simulink model "Ring_modulator"  (Simulink 10.0)
settings: Solver=ode45  StartTime=0.0  StopTime=10.0  RelTol=1e-3  EnableMultiTasking=on
settings Model: Creator=tjohnson  LastModifiedBy=unknown
settings DataIOCC: LimitDataPoints=on
settings DebuggingCC: UnderspecifiedInitializationDetection=Simplified  MergeDetectMultiDrivingBlocksExec=error
settings GRTTargetCC: GeneratePreprocessorConditionals=Disable all  CombineOutputUpdateFcns=on  GRTInterface=off
settings ConfigComp: CovExternalEMLEnable=off

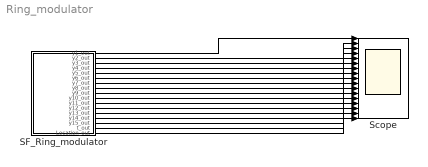
== system Ring_modulator ==
  SF_Ring_modulator : Stateflow chart  TreatAsAtomicUnit=on
  Scope : Scope  NumInputPorts=17
  wires:
  SF_Ring_modulator/1(y1_out) -> Scope/1
  SF_Ring_modulator/2(y2_out) -> Scope/2
  SF_Ring_modulator/3(y3_out) -> Scope/3
  SF_Ring_modulator/4(y4_out) -> Scope/4
  SF_Ring_modulator/5(y5_out) -> Scope/5
  SF_Ring_modulator/6(y6_out) -> Scope/6
  SF_Ring_modulator/7(y7_out) -> Scope/7
  SF_Ring_modulator/8(y8_out) -> Scope/8
  SF_Ring_modulator/9(y9_out) -> Scope/9
  SF_Ring_modulator/10(y10_out) -> Scope/10
  SF_Ring_modulator/11(y11_out) -> Scope/11
  SF_Ring_modulator/12(y12_out) -> Scope/12
  SF_Ring_modulator/13(y13_out) -> Scope/13
  SF_Ring_modulator/14(y14_out) -> Scope/14
  SF_Ring_modulator/15(y15_out) -> Scope/15
  SF_Ring_modulator/16(t_out) -> Scope/16
  SF_Ring_modulator/17(Location_out) -> Scope/17

== stateflow chart SF_Ring_modulator ==
  settings: updateMethod=CONTINUOUS
  state Ring_modulator
    du:
    y1_dot = 1.0 / C * (y8 - 0.5 * y10 + 0.5 * y11 + y14 - 1.0 / R * y1);
    y2_dot = 1.0 / C * (y9 - 0.5 * y12 + 0.5 * y13 + y15 - 1.0 / R * y2);
    y3_dot = 1.0 / Cs * (y10 - gamma * (exp(theta * (y3 - y5 - y7 - 2.0 * sin(20000.0 * pi * t))) - 1.0) + gamma * (exp(theta * (-y3 - y6 + y7 + 2.0 * sin(20000.0 * pi * t))) - 1.0));
    y4_dot = 1.0 / Cs * (-y11 + gamma * (exp(theta * (-y4 + y6 - y7 - 2.0 * sin(20000.0 * pi * t))) - 1.0) + gamma * (exp(theta * (y4 + y5 + y7 + 2.0 * sin(20000.0 * pi * t))) - 1.0));
    y5_dot = 1.0 / Cs * (y12 + gamma * (exp(theta * (y3 - y5 - y7 - 2.0 * sin(20000.0 * pi * t))) - 1.0) - gamma * (exp(theta * (y4 + y5 + y7 + 2.0 * sin(20000.0 * pi * t))) - 1.0));
    y6_dot = 1.0 / Cs * (-y13 - gamma * (exp(theta * (-y4 + y6 - y7 - 2.0 * sin(20000.0 * pi * t))) - 1.0) + gamma * (exp(theta * (-y3 - y6 + y7 + 2.0 * sin(20000.0 * pi * t))) - 1.0));
    y7_dot = 1.0 / Cp * (-(1.0 / Rp) * y7 + gamma * (exp(theta * (y3 - y5 - y7 - 2.0 * sin(20000.0 * pi * t))) - 1.0) + gamma * (exp(theta * (-y4 + y6 - y7 - 2.0 * sin(20000.0 * pi * t))) - 1.0) - gamma * (exp(theta * (y4 + y5 + y7 + 2.0 * sin(20000.0 * pi * t))) - 1.0) - gamma * (exp(theta * (-y3 - y6 + y7 + 2.0 * sin(20000.0 * pi * t))) - 1.0));
    y8_dot = -(1.0 / Lh) * y1;
    y9_dot = -(1.0 / Lh) * y2;
    y10_dot = 1.0 / Ls2 * (0.5 * y1 - y3 - Rg2 * y10);
    y11_dot = 1.0 / Ls3 * (-0.5 * y1 + y4 - Rg3 * y11);
    y12_dot = 1.0 / Ls2 * (0.5 * y2 - y5 - Rg2 * y12);
    y13_dot = 1.0 / Ls3 * (-0.5 * y2 + y6 - Rg3 * y13);
    y14_dot = 1.0 / Ls1 * (-y1 + 0.5 * sin(2000.0 * pi * t));
    y15_dot = 1.0 / Ls1 * (-y2 - (Rc + Rg1) * y15);
    t_dot = 1.0;
    y1_out=y1;
    y2_out=y2;
    y3_out=y3;
    y4_out=y4;
    y5_out=y5;
    y6_out=y6;
    y7_out=y7;
    y8_out=y8;
    y9_out=y9;
    y10_out=y10;
    y11_out=y11;
    y12_out=y12;
    y13_out=y13;
    y14_out=y14;
    y15_out=y15;
    t_out=t;
    Location_out =1;
  (default) -> Ring_modulator : {y1 = 0.0; y10 = 0.0; y11 = 0.0; y12 = 0.0; y13 = 0.0; y14 = 0.0; y15 = 0.0; y2 = 0.0; y3 = 0.0; y4 = 0.0; y5 = 0.0; y6 = 0.0; y7 = 0.0; y8 = 0.0; y9 = 0.0; C = 1.6E-7;}
  data: C constant double =1.6e-07; Cs constant double =2e-12; Cp constant double =1e-08; Lh constant double =4.45; Ls1 constant double =0.002; Ls2 constant double =0.0005; Ls3 constant double =0.0005; gamma constant double =4.0673e-08; R constant double =25000; Rp constant double =50; Rg1 constant double =36.3; Rg2 constant double =17.3; Rg3 constant double =17.3; Ri constant double =50; Rc constant double =600; theta constant double =17.7493; pi constant double =3.1416; y1 local double; y1_out output double; y2 local double; y2_out output double; y3 local double; y3_out output double; y4 local double; y4_out output double; y5 local double; y5_out output double; y6 local double; y6_out output double; y7 local double; y7_out output double; y8 local double; y8_out output double; y9 local double; y9_out output double; y10 local double; y10_out output double; y11 local double; y11_out output double; y12 local double; y12_out output double; y13 local double; y13_out output double; y14 local double; y14_out output double; y15 local double; y15_out output double; t local double; t_out output double; Location_out output double
  data y1 settings: updateMethod=SF_CONTINUOUS_TIME_DATA
  data y2 settings: updateMethod=SF_CONTINUOUS_TIME_DATA
  data y3 settings: updateMethod=SF_CONTINUOUS_TIME_DATA
  data y4 settings: updateMethod=SF_CONTINUOUS_TIME_DATA
  data y5 settings: updateMethod=SF_CONTINUOUS_TIME_DATA
  data y6 settings: updateMethod=SF_CONTINUOUS_TIME_DATA
  data y7 settings: updateMethod=SF_CONTINUOUS_TIME_DATA
  data y8 settings: updateMethod=SF_CONTINUOUS_TIME_DATA
  data y9 settings: updateMethod=SF_CONTINUOUS_TIME_DATA
  data y10 settings: updateMethod=SF_CONTINUOUS_TIME_DATA
  data y11 settings: updateMethod=SF_CONTINUOUS_TIME_DATA
  data y12 settings: updateMethod=SF_CONTINUOUS_TIME_DATA
  data y13 settings: updateMethod=SF_CONTINUOUS_TIME_DATA
  data y14 settings: updateMethod=SF_CONTINUOUS_TIME_DATA
  data y15 settings: updateMethod=SF_CONTINUOUS_TIME_DATA
  data t settings: updateMethod=SF_CONTINUOUS_TIME_DATA
